simulink model "HEMS_in_EV_Model"  (R2025b)
settings: Solver=ode4  StartTime=0.0  StopTime=3000  FixedStep=0.01  RelTol=1e-3  AbsTol=1e-3
libraries: fl_lib x8, nesl_utility x7, eeGeneralControl x1, simulink x1
settings Model: Creator=arani  LastModifiedBy=arani
settings SolverCC: AutoScaleAbsTol=off  AlgebraicLoopSolver=TrustRegion  MaxZcPerStep=1.0
settings DebuggingCC: UnconnectedInputMsg=warning  UnconnectedOutputMsg=warning  UnconnectedLineMsg=warning  SymbolicDimsDataTypeCodeGenerationDiagnostic=none
settings ModelReferenceCC: EnableRefExpFcnMdlSchedulingChecks=on
settings SFSimCC: CustomCodeUndefinedFunction=UseInterfaceOnly
settings RTWCC: GPUComputeCapability=3.5  DLArmComputeVersion=19.05
settings SimscapeCC: SimscapeLogType=all  SimscapeLogSimulationStatistics=on  SimscapeLogDataHistory=10000.0

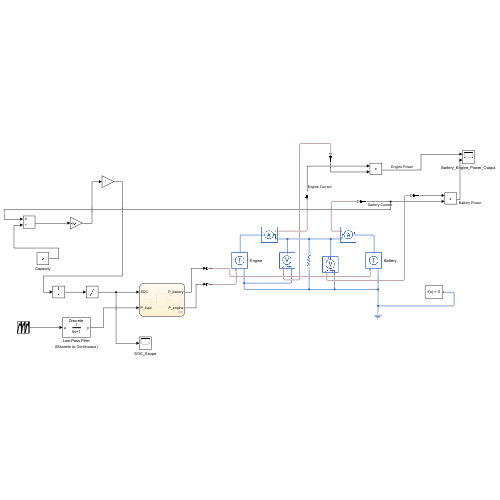
[thumbnail: Simulink's stored preview of the top-level diagram]
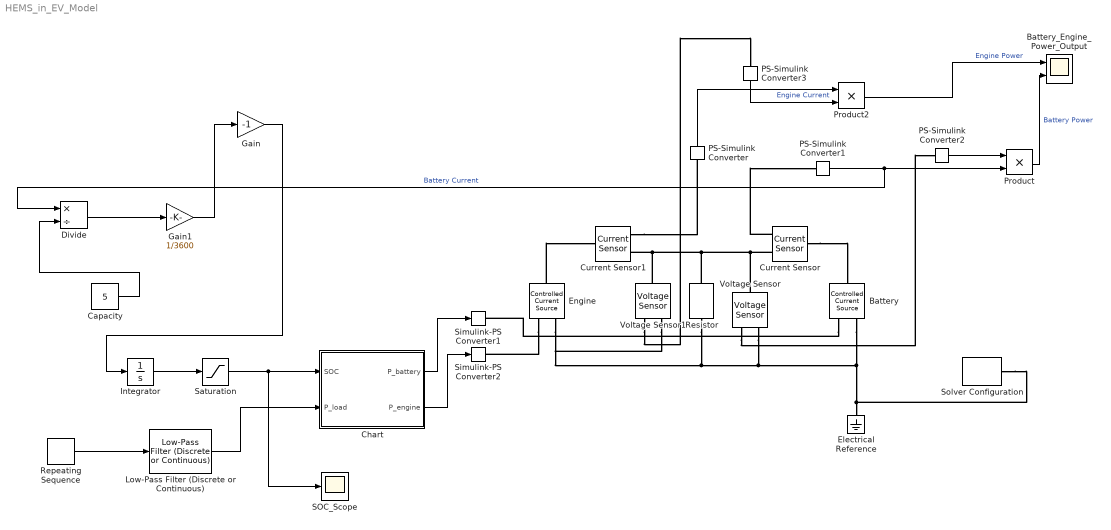
== system HEMS_in_EV_Model ==
  Battery : fl_lib/Electrical/Electrical Sources/Controlled Current Source
  Battery_Engine_Power_Output : Scope  NumInputPorts=2
      settings: ActiveDisplayYMinimum=-4.810328457686957E+6  ActiveDisplayYMaximum=5.87606379281542E+6
  Capacity : Constant  Value=5
  Chart : Stateflow chart  TreatAsAtomicUnit=on
  Current Sensor : fl_lib/Electrical/Electrical Sensors/Current Sensor
  Current Sensor1 : fl_lib/Electrical/Electrical Sensors/Current Sensor
  Divide : Product  Inputs=*/
  Electrical Reference : fl_lib/Electrical/Electrical Elements/Electrical Reference
  Engine : fl_lib/Electrical/Electrical Sources/Controlled Current Source
  Gain : Gain  Gain=-1
  Gain1 : Gain  Gain=1/3600
  Integrator : Integrator  InitialCondition=80
  Low-Pass Filter (Discrete or Continuous) : eeGeneralControl/Low-Pass Filter (Discrete or Continuous)  K=1  T=5  B=inf  A=-inf  init_option=Inherited from block input  x0=0  Ts=-1
  PS-Simulink Converter{,1..3} (4 alike) : nesl_utility/PS-Simulink Converter  PhysicalDomain=network_engine_domain  SubClassName=ps_output  LeftPortType=input  RightPortType=output  PseudoPeriodic=off  Frequencies=[]  VectorFormat=inherit  Unit=inherit  AffineConversion=off
  Product : Product
  Product2 : Product
  Repeating Sequence : simulink/Sources/Repeating Sequence  rep_seq_t=[0 5 10 15 20]  rep_seq_y=[1000 1500 2000 1800 2200]
  Resistor : fl_lib/Electrical/Electrical Elements/Resistor  R=1 Ohm  i_specify=off  i_priority=None  i=0 A  i_nominal_specify=off  i_nominal_value=1  i_nominal_unit=A  v_specify=off  v_priority=None  v=0 V  v_nominal_specify=off  v_nominal_value=1  v_nominal_unit=V
  SOC_Scope : Scope
      settings: ActiveDisplayYMinimum=-1  ActiveDisplayYMaximum=1  DataLoggingVariableName=ScopeData2
  Saturation : Saturate  UpperLimit=100  LowerLimit=0
  Simulink-PS Converter1 : nesl_utility/Simulink-PS Converter  PhysicalDomain=network_engine_domain  SubClassName=ps_input  LeftPortType=input  RightPortType=output  PseudoPeriodic=off  Frequencies=[]  NoiseDistribution=none  NoiseParameters=[]  Unit=A  AffineConversion=off  FilteringAndDerivatives=provide  SimscapeFilterOrder=1  InputFilterTimeConstant=0.001  UdotUserProvided=0
  Simulink-PS Converter2 : nesl_utility/Simulink-PS Converter  PhysicalDomain=network_engine_domain  SubClassName=ps_input  LeftPortType=input  RightPortType=output  PseudoPeriodic=off  Frequencies=[]  NoiseDistribution=none  NoiseParameters=[]  Unit=A  AffineConversion=off  FilteringAndDerivatives=provide  SimscapeFilterOrder=1  InputFilterTimeConstant=0.001  UdotUserProvided=0
  Solver Configuration : nesl_utility/Solver Configuration  PhysicalDomain=network_engine_domain  SubClassName=solver  LeftPortType=input  RightPortType=generic  Tones=[]  Harmonics=[]  SimulateNoise=off  Profile=off  UseLocalSampling=off  EnableSwitchedLinearOptims=on  FrequencyDomain=off  UseCCode=off  RelTol=0.001  AbsTol=0.001  MinStep=1e-09  ToWorkspace=off  RevertToSquareIcSolve=off  NumHomotopyIterations=100  PhasorMode=off  PhasorModeNumHarmonics=1  ConsistencySolver=NEWTON_XTOL_AFTER_FTOL  IndexReductionMethod=DerivativeReplacement  DoDC=off  ResidualTolerance=1e-09  ConsistencyTolSource=GLOBAL  ConsistencyAbsTol=0.001  ConsistencyRelTol=0.001  ConsistencyTolFactor=0.001  UseLocalSolver=off  LocalSolverChoice=NE_BACKWARD_EULER_ADVANCER  ResolveIndetEquations=on  FunctionEvalNumThread=1  LocalSolverSampleTime=0.001  DoFixedCost=off  MaxNonlinIter=3  MaxModeIter=2  ComputeImpulses=off  ImpulseIterations=2  LinearAlgebra=auto  LinearAlgebraNumThread=0  EquationFormulation=NE_TIME_EF  DelaysMemoryBudget=1024  AutomaticFiltering=on  FilteringTimeConstant=0.001  PartitionStorageMethod=AS_NEEDED  PartitionMemoryBudget=1024  PartitionMethod=ROBUST  MultibodyUseLocalSolver=off  MultibodyLocalSolverChoice=ODE1  MultibodyLocalSolverSampleTime=0.001
  Voltage Sensor : fl_lib/Electrical/Electrical Sensors/Voltage Sensor
  Voltage Sensor1 : fl_lib/Electrical/Electrical Sensors/Voltage Sensor
  wires:
  Chart/1(P_battery) -> Simulink-PS Converter1/1
  Chart/2(P_engine) -> Simulink-PS Converter2/1
  PS-Simulink Converter2/1 -> Product/1
  PS-Simulink Converter1/1 -> Divide/1, Product/2  "Battery Current"
  Product/1 -> Battery_Engine_Power_Output/2  "Battery Power"
  PS-Simulink Converter/1 -> Product2/1  "Engine Current"
  Product2/1 -> Battery_Engine_Power_Output/1  "Engine Power"
  Gain/1 -> Integrator/1
  Integrator/1 -> Saturation/1
  Saturation/1 -> SOC_Scope/1, Chart/1(SOC)
  Divide/1 -> Gain1/1
  Gain1/1 -> Gain/1
  PS-Simulink Converter3/1 -> Product2/2
  Repeating Sequence/1 -> Low-Pass Filter (Discrete or Continuous)/1
  Low-Pass Filter (Discrete or Continuous)/1 -> Chart/2(P_load)
  Capacity/1 -> Divide/2
  connections:
  Electrical Reference/LConn1 -- Voltage Sensor/RConn2 -- Resistor/RConn1 -- Voltage Sensor1/RConn2 -- Engine/RConn2 -- Battery/RConn2 -- Solver Configuration/RConn1
  Battery/RConn1 -- Simulink-PS Converter1/RConn1
  Engine/RConn1 -- Simulink-PS Converter2/RConn1
  Engine/LConn1 -- Current Sensor1/LConn1
  Current Sensor1/RConn1 -- PS-Simulink Converter/LConn1
  Current Sensor/LConn1 -- Battery/LConn1
  Current Sensor/RConn2 -- Voltage Sensor/LConn1 -- Resistor/LConn1 -- Voltage Sensor1/LConn1 -- Current Sensor1/RConn2
  Current Sensor/RConn1 -- PS-Simulink Converter1/LConn1
  Voltage Sensor/RConn1 -- PS-Simulink Converter2/LConn1
  Voltage Sensor1/RConn1 -- PS-Simulink Converter3/LConn1

== stateflow chart HEMS_in_EV_Model/Chart ==
  state Hybrid
    during:
    P_batt_max = 1500;
    % smoothing factor (0.1 = very smooth, 0.3 = faster response)
    k = 0.2;
    % target battery power based on SOC and load
    P_batt_target = min(P_batt_max * (SOC/100), P_load);
    % smooth transition (no step jump)
    P_battery = (1 - k) * P_battery + k * P_batt_target;
    % engine supplies remaining
    P_engine = P_load - P_battery;
    P_engine = max(0, P_engine);
  state Engine
    during:
    P_batt_max = 1500;
    % smoothing factor (keep same as Hybrid)
    k = 0.2;
    % reduced battery assist at low SOC
    P_batt_target = min(P_batt_max * (SOC/100), P_load);
    % smooth update (no sudden drop)
    P_battery = (1 - k) * P_battery + k * P_batt_target;
    % engine supplies the rest
    P_engine = P_load - P_battery;
    P_engine = max(0, P_engine);
  state Battery
    during:
    P_batt_max = 1500;
    if P_load <= P_batt_max
    P_battery = P_load;
    P_engine  = 0;
    else
    P_battery = P_batt_max;
    P_engine  = P_load - P_battery;
    end
  (default) -> Battery
  Hybrid -> Engine [order 1] : [ SOC <= 30 && after(1, sec) ]
  Engine -> Hybrid : [ SOC > 35 && after(1, sec) ]
  Battery -> Hybrid : [SOC < 60 && P_load > 1500 && after(1, sec)]
  Hybrid -> Battery [order 2] : [ SOC > 65 && after(1, sec) ]
  data: SOC input; P_load input; P_battery output; P_engine output; P_batt_max local; P_batt_target local; k local
